simulink model "tank"  (R2019b)
settings: Solver=ode45  StartTime=0.0  StopTime=inf  RelTol=1e-3  EnableMultiTasking=on
model workspace (MAT data in the model file):
  PLC_IP_Address = 'localhost'
libraries: sh_lib x74, nesl_utility x46, fl_lib x40, dspnetwork x33
(part 1 of 3)
settings Model: EnablePacing=on  PacingRate=0.100000  Creator=Rishabh  LastModifiedBy=jrsma
settings DataIOCC: LimitDataPoints=on  SaveFormat=Array  SignalLoggingSaveFormat=ModelDataLogs  ReturnWorkspaceOutputs=off
settings OptimizationCC: ExpressionDepthLimit=2147483647  InitFltsAndDblsToZero=on  LifeSpan=inf
settings DebuggingCC: UnderspecifiedInitializationDetection=Classic  MergeDetectMultiDrivingBlocksExec=none  SolverPrmCheckMsg=warning  FcnCallInpInsideContextMsg=warning  AllowSymbolicDim=off  StateNameClashWarn=warning  SFUnexpectedBacktrackingDiag=warning  SFNoUnconditionalDefaultTransitionDiag=warning  SFExecutionAtInitializationDiag=none  ArithmeticOperatorsInVariantConditions=warning
settings HardwareCC: ProdBitPerPointer=32  ProdBitPerSizeT=32  ProdBitPerPtrDiffT=32  ProdLargestAtomicFloat=None  ProdIntDivRoundTo=Undefined  ProdEndianess=Unspecified  ProdWordSize=32  ProdHWDeviceType=32-bit Generic
settings ModelReferenceCC: PropagateSignalLabelsOutOfModel=off
settings SFSimCC: SimUseLocalCustomCode=off  CustomCodeUndefinedFunction=UseInterfaceOnly
settings RTWCC: RTWUseLocalCustomCode=off
settings CodeAppCC: StateflowObjectComments=on
settings GRTTargetCC: TargetLangStandard=C89/C90 (ANSI)  CombineOutputUpdateFcns=off  GRTInterface=on
settings ConfigComp: CovMetricSettings=dw  CovHtmlReporting=on  CovSaveCumulativeToWorkspaceVar=on  CovSaveSingleToWorkspaceVar=on  CovExternalEMLEnable=off
settings SimscapeCC: SimscapeNormalizeSystem=off

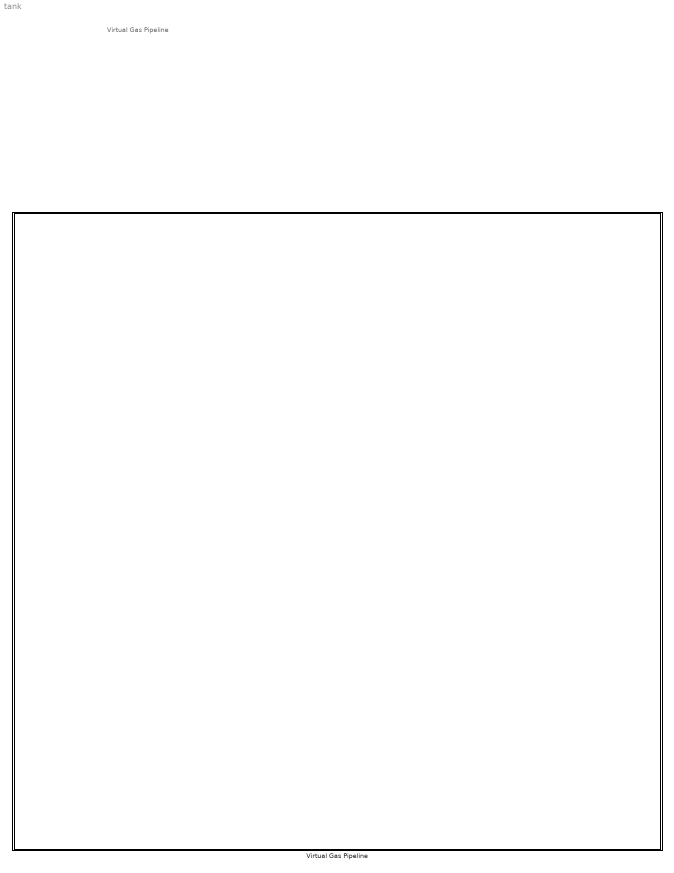
== system tank ==
  note: Virtual Gas Pipeline
  "Virtual Gas Pipeline " : Subsystem

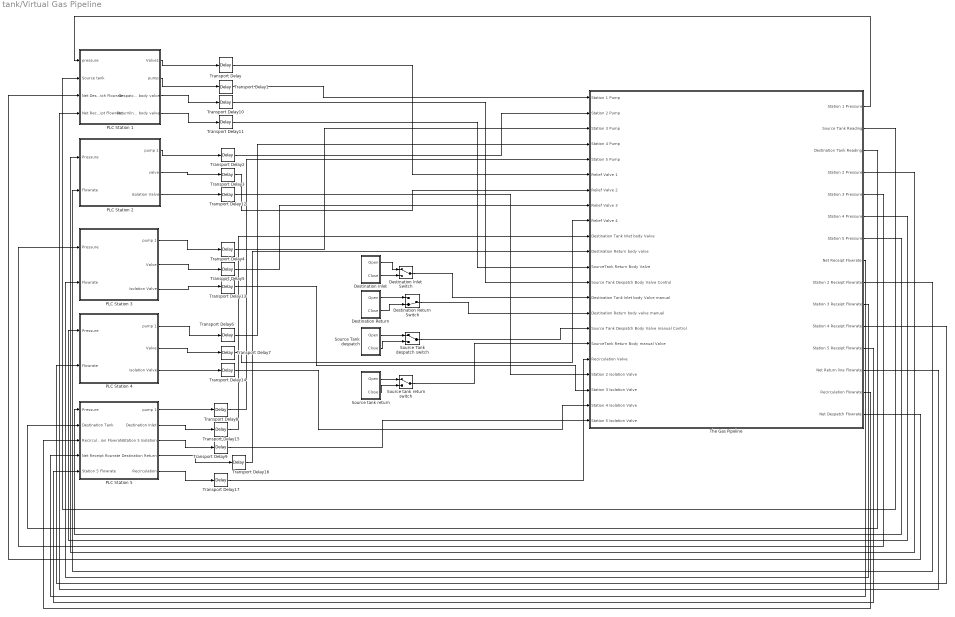
== system tank/Virtual Gas Pipeline  ==
  "  PLC Station 2" : Subsystem  TreatAsAtomicUnit=on
  " PLC Station 1" : Subsystem  TreatAsAtomicUnit=on
  Destination Inlet : Subsystem
  Destination Inlet Switch : ManualSwitch
  Destination Return : Subsystem
  Destination Return Switch : ManualSwitch  CurrentSetting=0
  PLC Station 3 : Subsystem  TreatAsAtomicUnit=on
  PLC Station 4 : Subsystem  TreatAsAtomicUnit=on
  PLC Station 5 : Subsystem  TreatAsAtomicUnit=on
  Source Tank despatch : Subsystem
  Source Tank despatch switch : ManualSwitch
  "Source tank return " : Subsystem
  Source tank return switch : ManualSwitch
  The Gas Pipeline : Subsystem
  Transport Delay{,1..17} (18 alike) : TransportDelay  DelayTime=0.00002
  wires:
  The Gas Pipeline/1(Station 1 Pressure) -> " PLC Station 1"/1(pressure)
  PLC Station 3/1(pump 1) -> Transport Delay4/1
  PLC Station 3/2(Valve) -> Transport Delay5/1
  "  PLC Station 2"/2(valve) -> Transport Delay3/1
  PLC Station 4/2(Valve) -> Transport Delay7/1
  PLC Station 5/1(pump 1) -> Transport Delay8/1
  "  PLC Station 2"/1(pump 1) -> Transport Delay2/1
  " PLC Station 1"/2("pump ") -> Transport Delay1/1
  " PLC Station 1"/1(Valve1) -> Transport Delay/1
  PLC Station 4/1(pump 1) -> Transport Delay6/1
  The Gas Pipeline/2(Source Tank Reading) -> " PLC Station 1"/2(Source tank)
  The Gas Pipeline/3(Destination Tank Reading) -> PLC Station 5/2(Destination Tank)
  Destination Inlet/1(Open) -> Destination Inlet Switch/1
  Destination Inlet/2("Close ") -> Destination Inlet Switch/2
  Destination Inlet Switch/1 -> The Gas Pipeline/14(Destination Tank Inlet body Valve manual)
  Destination Return/1(Open) -> Destination Return Switch/1
  Destination Return/2(Close) -> Destination Return Switch/2
  Destination Return Switch/1 -> The Gas Pipeline/15(Destination Return body valve manual)
  Source Tank despatch/1(Open) -> Source Tank despatch switch/1
  Source Tank despatch/2(Close) -> Source Tank despatch switch/2
  Source Tank despatch switch/1 -> The Gas Pipeline/16(Source Tank Despatch Body Valve manual Control)
  "Source tank return "/1(Open) -> Source tank return switch/1
  "Source tank return "/2(Close) -> Source tank return switch/2
  Source tank return switch/1 -> The Gas Pipeline/17(SourceTank Return Body manual Valve)
  The Gas Pipeline/7(Station 5 Pressure) -> PLC Station 5/1("Pressure ")
  The Gas Pipeline/6(Station 4 Pressure) -> PLC Station 4/1("Pressure ")
  The Gas Pipeline/5(Station 3 Pressure) -> PLC Station 3/1("Pressure ")
  The Gas Pipeline/4(Station 2 Pressure) -> "  PLC Station 2"/1(Pressure)
  Transport Delay/1 -> The Gas Pipeline/6(Relief Valve 1)
  Transport Delay1/1 -> The Gas Pipeline/1(Station 1 Pump)
  Transport Delay2/1 -> The Gas Pipeline/2("Station 2 Pump ")
  Transport Delay3/1 -> The Gas Pipeline/7(Relief Valve 2)
  Transport Delay4/1 -> The Gas Pipeline/3("Station 3 Pump ")
  Transport Delay5/1 -> The Gas Pipeline/8(Relief Valve 3)
  Transport Delay6/1 -> The Gas Pipeline/4("Station 4 Pump ")
  Transport Delay8/1 -> The Gas Pipeline/5(Station 5 Pump)
  Transport Delay7/1 -> The Gas Pipeline/9(Relief Valve 4)
  The Gas Pipeline/15(Net Despatch Flowrate) -> " PLC Station 1"/3(Net Despatch Flowrate)
  The Gas Pipeline/9(Station 2 Receipt Flowrate) -> "  PLC Station 2"/2(Flowrate)
  The Gas Pipeline/10(Station 3 Receipt Flowrate) -> PLC Station 3/2(Flowrate)
  The Gas Pipeline/11(Station 4 Receipt Flowrate) -> PLC Station 4/2(Flowrate)
  The Gas Pipeline/13(Net Return line Flowrate) -> " PLC Station 1"/4(Net Receipt Flowrate)
  " PLC Station 1"/3(Despatch body valve) -> Transport Delay10/1
  " PLC Station 1"/4(Returnline body valve) -> Transport Delay11/1
  Transport Delay10/1 -> The Gas Pipeline/13(Source Tank Despatch Body Valve Control)
  Transport Delay11/1 -> The Gas Pipeline/12(SourceTank Return Body Valve)
  "  PLC Station 2"/3(Isolation Valve) -> Transport Delay12/1
  Transport Delay12/1 -> The Gas Pipeline/19(Station 2 Isolation Valve)
  PLC Station 3/3(Isolation Valve) -> Transport Delay13/1
  Transport Delay13/1 -> The Gas Pipeline/20(Station 3 Isolation Valve)
  PLC Station 4/3(Isolation Valve) -> Transport Delay14/1
  Transport Delay14/1 -> The Gas Pipeline/21(Station 4 Isolation Valve)
  The Gas Pipeline/8(Net Receipt Flowrate) -> PLC Station 5/4(Net Receipt flowrate)
  The Gas Pipeline/12(Station 5 Receipt Flowrate) -> PLC Station 5/5(Station 5 Flowrate)
  The Gas Pipeline/14(Recirculation Flowrate) -> PLC Station 5/3(Recirculation Flowrate)
  PLC Station 5/2(Destination Inlet) -> Transport Delay15/1
  PLC Station 5/3(Station 5 Isolation) -> Transport Delay9/1
  PLC Station 5/4(Destination Return) -> Transport Delay16/1
  PLC Station 5/5(Recirculation) -> Transport Delay17/1
  Transport Delay15/1 -> The Gas Pipeline/10(Destination Tank Inlet body Valve)
  Transport Delay9/1 -> The Gas Pipeline/22(Station 5 Isolation Valve)
  Transport Delay16/1 -> The Gas Pipeline/11(Destination Return body valve)
  Transport Delay17/1 -> The Gas Pipeline/18(Recirculation Valve)

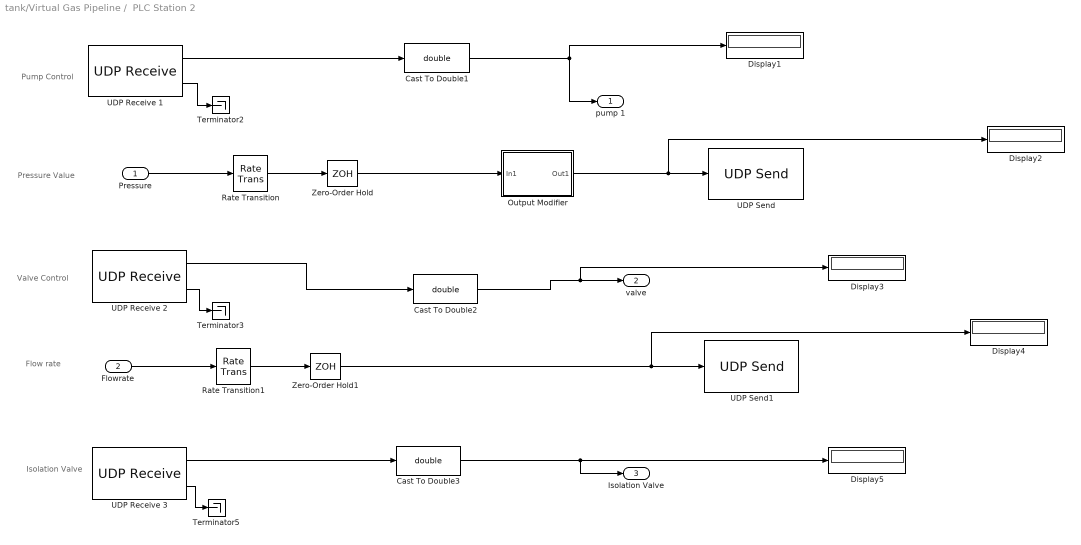
== system tank/Virtual Gas Pipeline /  PLC Station 2 ==
  note: Isolation Valve
  note: Flow rate
  note: Valve Control
  note: Pump Control
  note: Pressure Value
  Pressure : Inport
  Flowrate : Inport  Port=2
  Cast To Double1 : DataTypeConversion  OutDataTypeStr=double
  Cast To Double2 : DataTypeConversion  OutDataTypeStr=double
  Cast To Double3 : DataTypeConversion  OutDataTypeStr=double
  Display{1..5} (5 alike) : Display
  Output Modifier : Subsystem
  Rate Transition : RateTransition
  Rate Transition1 : RateTransition
  Terminator2 : Terminator
  Terminator3 : Terminator
  Terminator5 : Terminator
  UDP Receive 1 : dspnetwork/UDP Receive  localURL='0.0.0.0'  localPort=20001  remoteURL='0.0.0.0'  remotePort=-1  recvBufferSize=2  dims=1  signalDatatype=uint16  isComplex=off  isVarSize=off  showBlockingTime=on  blockingTime=0  sampletime=0.01  blockPlatform=LINUX
      settings: SourceProductName=Simulink
  UDP Receive 2 : dspnetwork/UDP Receive  localURL='0.0.0.0'  localPort=20003  remoteURL='0.0.0.0'  remotePort=-1  recvBufferSize=2  dims=1  signalDatatype=uint16  isComplex=off  isVarSize=off  showBlockingTime=on  blockingTime=0  sampletime=0.01  blockPlatform=LINUX
      settings: SourceProductName=Simulink
  UDP Receive 3 : dspnetwork/UDP Receive  localURL='0.0.0.0'  localPort=20005  remoteURL='0.0.0.0'  remotePort=-1  recvBufferSize=2  dims=1  signalDatatype=uint16  isComplex=off  isVarSize=off  showBlockingTime=on  blockingTime=0  sampletime=0.01  blockPlatform=LINUX
      settings: SourceProductName=Simulink
  UDP Send : dspnetwork/UDP Send  remoteURL=PLC_IP_Address  remotePort=20002  localURL='255.255.255.255'  localPortSource=Automatically determine  localPort=-1  sampletime=-1  blockPlatform=LINUX  separateLengthPort=0
      settings: SourceProductName=Simulink
  UDP Send1 : dspnetwork/UDP Send  remoteURL=PLC_IP_Address  remotePort=20004  localURL='255.255.255.255'  localPortSource=Automatically determine  localPort=-1  sampletime=-1  blockPlatform=LINUX  separateLengthPort=0
      settings: SourceProductName=Simulink
  Zero-Order Hold : ZeroOrderHold  SampleTime=0.1
  Zero-Order Hold1 : ZeroOrderHold  SampleTime=0.1
  pump 1 : Outport  PortDimensions=1
  valve : Outport  Port=2  PortDimensions=1
  Isolation Valve : Outport  Port=3  PortDimensions=1
  wires:
  UDP Receive 1/2 -> Terminator2/1
  UDP Receive 2/1 -> Cast To Double2/1
  UDP Receive 2/2 -> Terminator3/1
  Cast To Double2/1 -> Display3/1, valve/1
  Rate Transition/1 -> Zero-Order Hold/1
  Pressure/1 -> Rate Transition/1
  Cast To Double1/1 -> pump 1/1, Display1/1
  Zero-Order Hold/1 -> Output Modifier/1(In1)
  Output Modifier/1(Out1) -> Display2/1, UDP Send/1
  Rate Transition1/1 -> Zero-Order Hold1/1
  Flowrate/1 -> Rate Transition1/1
  Zero-Order Hold1/1 -> Display4/1, UDP Send1/1
  UDP Receive 3/1 -> Cast To Double3/1
  UDP Receive 3/2 -> Terminator5/1
  Cast To Double3/1 -> Isolation Valve/1, Display5/1
  UDP Receive 1/1 -> Cast To Double1/1

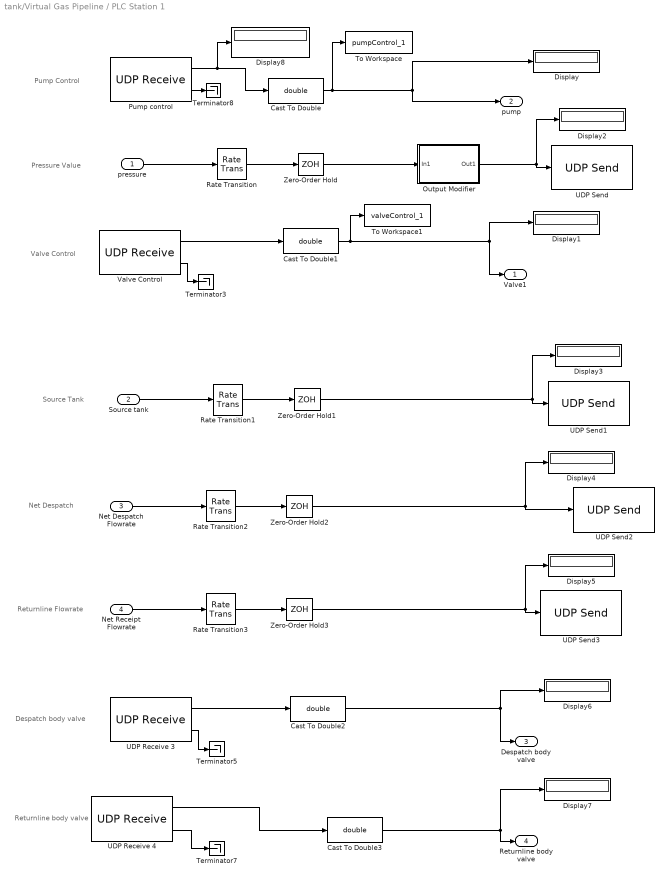
== system tank/Virtual Gas Pipeline / PLC Station 1 ==
  note: Despatch body valve
  note: Returnline body valve
  note: Returnline Flowrate
  note: Net Despatch
  note: Source Tank
  note: Valve Control
  note: Pump Control
  note: Pressure Value
  pressure : Inport
  Source tank : Inport  Port=2
  Net Despatch Flowrate : Inport  Port=3
  Net Receipt Flowrate : Inport  Port=4
  Cast To Double{,1..3} (4 alike) : DataTypeConversion  OutDataTypeStr=double
  Display{,1..8} (9 alike) : Display
  Output Modifier : Subsystem
  Pump control : dspnetwork/UDP Receive  localURL='0.0.0.0'  localPort=10001  remoteURL='0.0.0.0'  remotePort=-1  recvBufferSize=2  dims=1  signalDatatype=uint16  isComplex=off  isVarSize=off  showBlockingTime=on  blockingTime=0  sampletime=0.01  blockPlatform=LINUX
      settings: SourceProductName=Simulink
  Rate Transition{,1..3} (4 alike) : RateTransition
  Terminator{3,5,7..8} (4 alike) : Terminator
  To Workspace : ToWorkspace  VariableName=pumpControl_1  SaveFormat=Timeseries  SampleTime=-1
  To Workspace1 : ToWorkspace  VariableName=valveControl_1  SaveFormat=Timeseries  SampleTime=-1
  UDP Receive 3 : dspnetwork/UDP Receive  localURL='0.0.0.0'  localPort=10007  remoteURL='0.0.0.0'  remotePort=-1  recvBufferSize=2  dims=1  signalDatatype=uint16  isComplex=off  isVarSize=off  showBlockingTime=on  blockingTime=0  sampletime=0.01  blockPlatform=LINUX
      settings: SourceProductName=Simulink
  UDP Receive 4 : dspnetwork/UDP Receive  localURL='0.0.0.0'  localPort=10008  remoteURL='0.0.0.0'  remotePort=-1  recvBufferSize=2  dims=1  signalDatatype=uint16  isComplex=off  isVarSize=off  showBlockingTime=on  blockingTime=0  sampletime=0.01  blockPlatform=LINUX
      settings: SourceProductName=Simulink
  UDP Send : dspnetwork/UDP Send  remoteURL=PLC_IP_Address  remotePort=10002  localURL='255.255.255.255'  localPortSource=Automatically determine  localPort=-1  sampletime=-1  blockPlatform=LINUX  separateLengthPort=0
      settings: SourceProductName=Simulink
  UDP Send1 : dspnetwork/UDP Send  remoteURL=PLC_IP_Address  remotePort=10004  localURL='255.255.255.255'  localPortSource=Automatically determine  localPort=-1  sampletime=-1  blockPlatform=LINUX  separateLengthPort=0
      settings: SourceProductName=Simulink
  UDP Send2 : dspnetwork/UDP Send  remoteURL=PLC_IP_Address  remotePort=10005  localURL='255.255.255.255'  localPortSource=Automatically determine  localPort=-1  sampletime=-1  blockPlatform=LINUX  separateLengthPort=0
      settings: SourceProductName=Simulink
  UDP Send3 : dspnetwork/UDP Send  remoteURL=PLC_IP_Address  remotePort=10006  localURL='255.255.255.255'  localPortSource=Automatically determine  localPort=-1  sampletime=-1  blockPlatform=LINUX  separateLengthPort=0
      settings: SourceProductName=Simulink
  Valve Control : dspnetwork/UDP Receive  localURL='0.0.0.0'  localPort=10003  remoteURL='0.0.0.0'  remotePort=-1  recvBufferSize=2  dims=1  signalDatatype=uint16  isComplex=off  isVarSize=off  showBlockingTime=on  blockingTime=0  sampletime=0.01  blockPlatform=LINUX
      settings: SourceProductName=Simulink
  Zero-Order Hold{,1..3} (4 alike) : ZeroOrderHold  SampleTime=0.1
  Valve1 : Outport  PortDimensions=1
  "pump " : Outport  Port=2  PortDimensions=1
  Despatch body valve : Outport  Port=3  PortDimensions=1
  Returnline body valve : Outport  Port=4  PortDimensions=1
  wires:
  Valve Control/1 -> Cast To Double1/1
  Valve Control/2 -> Terminator3/1
  Rate Transition/1 -> Zero-Order Hold/1
  pressure/1 -> Rate Transition/1
  Cast To Double1/1 -> To Workspace1/1, Valve1/1, Display1/1
  Output Modifier/1(Out1) -> UDP Send/1, Display2/1
  Zero-Order Hold/1 -> Output Modifier/1(In1)
  Rate Transition1/1 -> Zero-Order Hold1/1
  Source tank/1 -> Rate Transition1/1
  Zero-Order Hold1/1 -> Display3/1, UDP Send1/1
  Rate Transition2/1 -> Zero-Order Hold2/1
  Net Despatch Flowrate/1 -> Rate Transition2/1
  Zero-Order Hold2/1 -> Display4/1, UDP Send2/1
  Rate Transition3/1 -> Zero-Order Hold3/1
  Net Receipt Flowrate/1 -> Rate Transition3/1
  Zero-Order Hold3/1 -> Display5/1, UDP Send3/1
  UDP Receive 3/1 -> Cast To Double2/1
  UDP Receive 3/2 -> Terminator5/1
  Cast To Double2/1 -> Despatch body valve/1, Display6/1
  UDP Receive 4/2 -> Terminator7/1
  Cast To Double3/1 -> Returnline body valve/1, Display7/1
  Pump control/2 -> Terminator8/1
  Pump control/1 -> Cast To Double/1, Display8/1
  Cast To Double/1 -> To Workspace/1, Display/1, "pump "/1
  UDP Receive 4/1 -> Cast To Double3/1

== system tank/Virtual Gas Pipeline /Destination Inlet ==
  Constant : Constant
  Constant1 : Constant  Value=0
  Open : Outport
  "Close " : Outport  Port=2
  wires:
  Constant1/1 -> "Close "/1
  Constant/1 -> Open/1

== system tank/Virtual Gas Pipeline /Destination Return ==
  Constant : Constant
  Constant1 : Constant  Value=0
  Open : Outport
  Close : Outport  Port=2
  wires:
  Constant1/1 -> Close/1
  Constant/1 -> Open/1

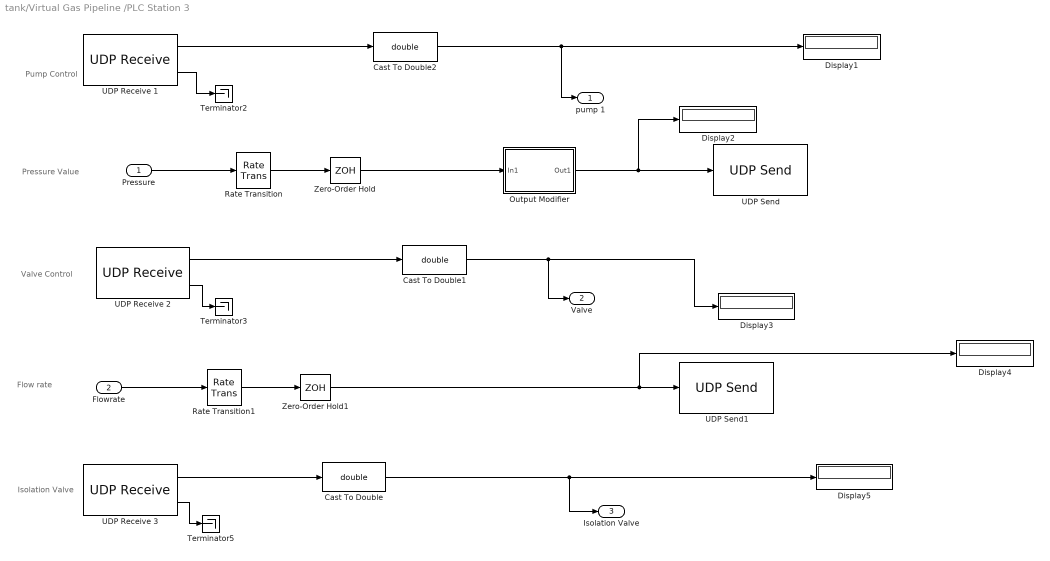
== system tank/Virtual Gas Pipeline /PLC Station 3 ==
  note: Valve Control
  note: Pump Control
  note: Pressure Value
  note: Isolation Valve
  note: Flow rate
  "Pressure " : Inport
  Flowrate : Inport  Port=2
  Cast To Double : DataTypeConversion  OutDataTypeStr=double
  Cast To Double1 : DataTypeConversion  OutDataTypeStr=double
  Cast To Double2 : DataTypeConversion  OutDataTypeStr=double
  Display{1..5} (5 alike) : Display
  Output Modifier : Subsystem
  Rate Transition : RateTransition
  Rate Transition1 : RateTransition
  Terminator2 : Terminator
  Terminator3 : Terminator
  Terminator5 : Terminator
  UDP Receive 1 : dspnetwork/UDP Receive  localURL='0.0.0.0'  localPort=30001  remoteURL='0.0.0.0'  remotePort=-1  recvBufferSize=2  dims=1  signalDatatype=uint16  isComplex=off  isVarSize=off  showBlockingTime=on  blockingTime=0  sampletime=0.01  blockPlatform=LINUX
      settings: SourceProductName=Simulink
  UDP Receive 2 : dspnetwork/UDP Receive  localURL='0.0.0.0'  localPort=30003  remoteURL='0.0.0.0'  remotePort=-1  recvBufferSize=2  dims=1  signalDatatype=uint16  isComplex=off  isVarSize=off  showBlockingTime=on  blockingTime=0  sampletime=0.01  blockPlatform=LINUX
      settings: SourceProductName=Simulink
  UDP Receive 3 : dspnetwork/UDP Receive  localURL='0.0.0.0'  localPort=30005  remoteURL='0.0.0.0'  remotePort=-1  recvBufferSize=2  dims=1  signalDatatype=uint16  isComplex=off  isVarSize=off  showBlockingTime=on  blockingTime=0  sampletime=0.01  blockPlatform=LINUX
      settings: SourceProductName=Simulink
  UDP Send : dspnetwork/UDP Send  remoteURL=PLC_IP_Address  remotePort=30002  localURL='255.255.255.255'  localPortSource=Automatically determine  localPort=-1  sampletime=-1  blockPlatform=LINUX  separateLengthPort=0
      settings: SourceProductName=Simulink
  UDP Send1 : dspnetwork/UDP Send  remoteURL=PLC_IP_Address  remotePort=30004  localURL='255.255.255.255'  localPortSource=Automatically determine  localPort=-1  sampletime=-1  blockPlatform=LINUX  separateLengthPort=0
      settings: SourceProductName=Simulink
  Zero-Order Hold : ZeroOrderHold  SampleTime=0.1
  Zero-Order Hold1 : ZeroOrderHold  SampleTime=0.1
  pump 1 : Outport  PortDimensions=1
  Valve : Outport  Port=2  PortDimensions=1
  Isolation Valve : Outport  Port=3  PortDimensions=1
  wires:
  UDP Receive 1/2 -> Terminator2/1
  UDP Receive 2/2 -> Terminator3/1
  Cast To Double1/1 -> Valve/1, Display3/1
  Cast To Double2/1 -> pump 1/1, Display1/1
  Rate Transition/1 -> Zero-Order Hold/1
  "Pressure "/1 -> Rate Transition/1
  Zero-Order Hold/1 -> Output Modifier/1(In1)
  Output Modifier/1(Out1) -> Display2/1, UDP Send/1
  Rate Transition1/1 -> Zero-Order Hold1/1
  Flowrate/1 -> Rate Transition1/1
  Zero-Order Hold1/1 -> Display4/1, UDP Send1/1
  UDP Receive 3/2 -> Terminator5/1
  Cast To Double/1 -> Isolation Valve/1, Display5/1
  UDP Receive 1/1 -> Cast To Double2/1
  UDP Receive 2/1 -> Cast To Double1/1
  UDP Receive 3/1 -> Cast To Double/1

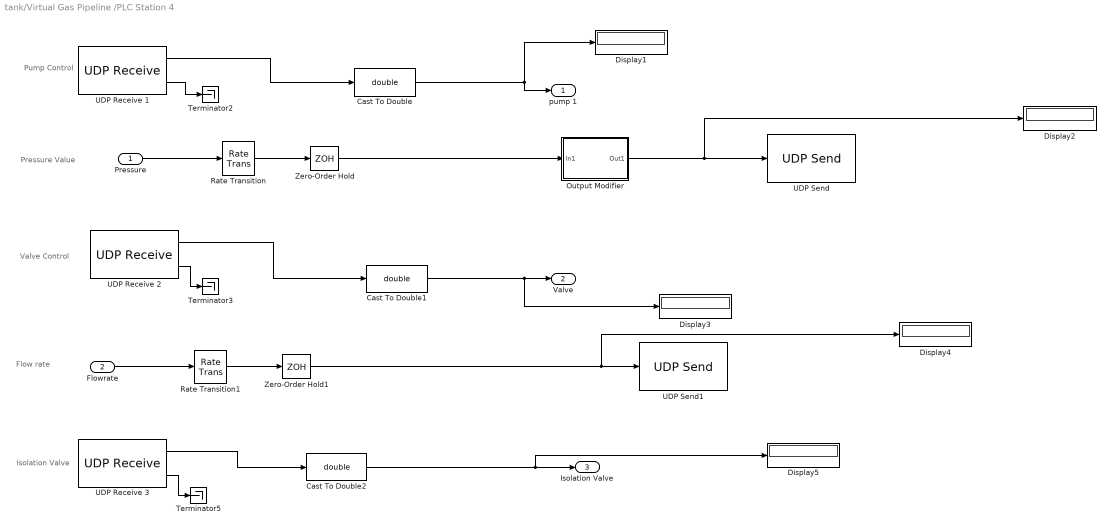
== system tank/Virtual Gas Pipeline /PLC Station 4 ==
  note: Valve Control
  note: Pump Control
  note: Pressure Value
  note: Isolation Valve
  note: Flow rate
  "Pressure " : Inport
  Flowrate : Inport  Port=2
  Cast To Double : DataTypeConversion  OutDataTypeStr=double
  Cast To Double1 : DataTypeConversion  OutDataTypeStr=double
  Cast To Double2 : DataTypeConversion  OutDataTypeStr=double
  Display{1..5} (5 alike) : Display
  Output Modifier : Subsystem
  Rate Transition : RateTransition
  Rate Transition1 : RateTransition
  Terminator2 : Terminator
  Terminator3 : Terminator
  Terminator5 : Terminator
  UDP Receive 1 : dspnetwork/UDP Receive  localURL='0.0.0.0'  localPort=40001  remoteURL='0.0.0.0'  remotePort=-1  recvBufferSize=2  dims=1  signalDatatype=uint16  isComplex=off  isVarSize=off  showBlockingTime=on  blockingTime=0  sampletime=0.01  blockPlatform=LINUX
      settings: SourceProductName=Simulink
  UDP Receive 2 : dspnetwork/UDP Receive  localURL='0.0.0.0'  localPort=40003  remoteURL='0.0.0.0'  remotePort=-1  recvBufferSize=2  dims=1  signalDatatype=uint16  isComplex=off  isVarSize=off  showBlockingTime=on  blockingTime=0  sampletime=0.01  blockPlatform=LINUX
      settings: SourceProductName=Simulink
  UDP Receive 3 : dspnetwork/UDP Receive  localURL='0.0.0.0'  localPort=40005  remoteURL='0.0.0.0'  remotePort=-1  recvBufferSize=2  dims=1  signalDatatype=uint16  isComplex=off  isVarSize=off  showBlockingTime=on  blockingTime=0  sampletime=0.01  blockPlatform=LINUX
      settings: SourceProductName=Simulink
  UDP Send : dspnetwork/UDP Send  remoteURL=PLC_IP_Address  remotePort=40002  localURL='255.255.255.255'  localPortSource=Automatically determine  localPort=-1  sampletime=-1  blockPlatform=LINUX  separateLengthPort=0
      settings: SourceProductName=Simulink
  UDP Send1 : dspnetwork/UDP Send  remoteURL=PLC_IP_Address  remotePort=40004  localURL='255.255.255.255'  localPortSource=Automatically determine  localPort=-1  sampletime=-1  blockPlatform=LINUX  separateLengthPort=0
      settings: SourceProductName=Simulink
  Zero-Order Hold : ZeroOrderHold  SampleTime=0.1
  Zero-Order Hold1 : ZeroOrderHold  SampleTime=0.1
  pump 1 : Outport  PortDimensions=1
  Valve : Outport  Port=2  PortDimensions=1
  Isolation Valve : Outport  Port=3  PortDimensions=1
  wires:
  UDP Receive 1/2 -> Terminator2/1
  UDP Receive 2/1 -> Cast To Double1/1
  UDP Receive 2/2 -> Terminator3/1
  Cast To Double1/1 -> Display3/1, Valve/1
  Cast To Double/1 -> pump 1/1, Display1/1
  UDP Receive 1/1 -> Cast To Double/1
  Rate Transition/1 -> Zero-Order Hold/1
  "Pressure "/1 -> Rate Transition/1
  Zero-Order Hold/1 -> Output Modifier/1(In1)
  Output Modifier/1(Out1) -> Display2/1, UDP Send/1
  Rate Transition1/1 -> Zero-Order Hold1/1
  Flowrate/1 -> Rate Transition1/1
  Zero-Order Hold1/1 -> Display4/1, UDP Send1/1
  UDP Receive 3/1 -> Cast To Double2/1
  UDP Receive 3/2 -> Terminator5/1
  Cast To Double2/1 -> Display5/1, Isolation Valve/1

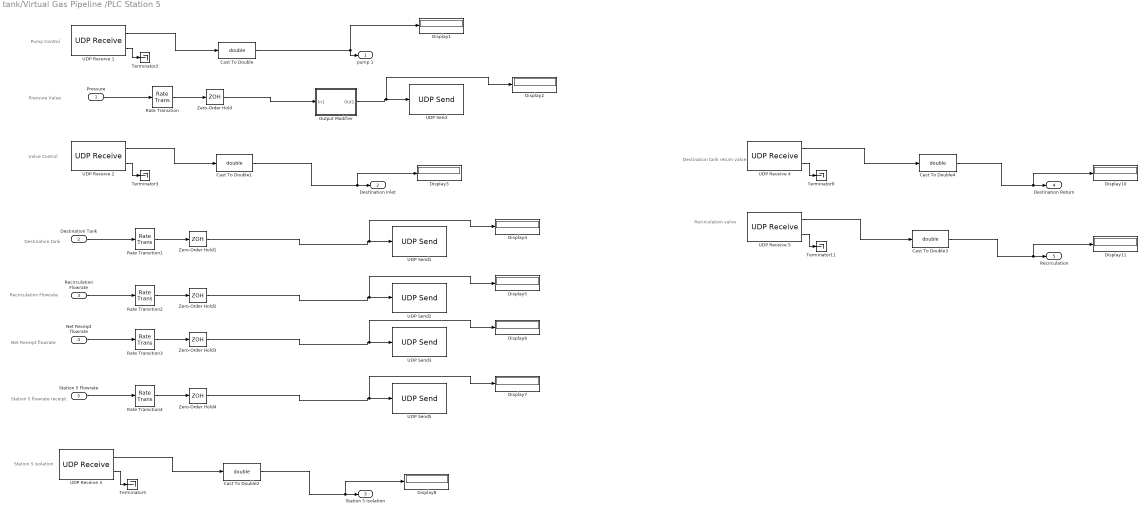
== system tank/Virtual Gas Pipeline /PLC Station 5 ==
  note: Recirculation valve
  note: Destination tank return valve
  note: Station 5 Isolation
  note: Net Receipt flowrate
  note: Recirculation Flowrate
  note: Destination tank
  note: Valve Control
  note: Pump Control
  note: Pressure Value
  note: Station 5 flowrate receipt
  "Pressure " : Inport
  Destination Tank : Inport  Port=2
  Recirculation Flowrate : Inport  Port=3
  Net Receipt flowrate : Inport  Port=4
  Station 5 Flowrate : Inport  Port=5
  Cast To Double{,1..4} (5 alike) : DataTypeConversion  OutDataTypeStr=double
  Display{1..8,10..11} (10 alike) : Display
  Output Modifier : Subsystem
  Rate Transition{,1..4} (5 alike) : RateTransition
  Terminator{2..3,5,9,11} (5 alike) : Terminator
  UDP Receive 1 : dspnetwork/UDP Receive  localURL='0.0.0.0'  localPort=50001  remoteURL='0.0.0.0'  remotePort=-1  recvBufferSize=2  dims=1  signalDatatype=uint16  isComplex=off  isVarSize=off  showBlockingTime=on  blockingTime=0  sampletime=0.01  blockPlatform=LINUX
      settings: SourceProductName=Simulink
  UDP Receive 2 : dspnetwork/UDP Receive  localURL='0.0.0.0'  localPort=50003  remoteURL='0.0.0.0'  remotePort=-1  recvBufferSize=2  dims=1  signalDatatype=uint16  isComplex=off  isVarSize=off  showBlockingTime=on  blockingTime=0  sampletime=0.01  blockPlatform=LINUX
      settings: SourceProductName=Simulink
  UDP Receive 3 : dspnetwork/UDP Receive  localURL='0.0.0.0'  localPort=50008  remoteURL='0.0.0.0'  remotePort=-1  recvBufferSize=2  dims=1  signalDatatype=uint16  isComplex=off  isVarSize=off  showBlockingTime=on  blockingTime=0  sampletime=0.01  blockPlatform=LINUX
      settings: SourceProductName=Simulink
  UDP Receive 4 : dspnetwork/UDP Receive  localURL='0.0.0.0'  localPort=5009  remoteURL='0.0.0.0'  remotePort=-1  recvBufferSize=2  dims=1  signalDatatype=uint16  isComplex=off  isVarSize=off  showBlockingTime=on  blockingTime=0  sampletime=0.01  blockPlatform=LINUX
      settings: SourceProductName=Simulink
  UDP Receive 5 : dspnetwork/UDP Receive  localURL='0.0.0.0'  localPort=50010  remoteURL='0.0.0.0'  remotePort=-1  recvBufferSize=2  dims=1  signalDatatype=uint16  isComplex=off  isVarSize=off  showBlockingTime=on  blockingTime=0  sampletime=0.01  blockPlatform=LINUX
      settings: SourceProductName=Simulink
  UDP Send : dspnetwork/UDP Send  remoteURL=PLC_IP_Address  remotePort=50002  localURL='255.255.255.255'  localPortSource=Automatically determine  localPort=-1  sampletime=-1  blockPlatform=LINUX  separateLengthPort=0
      settings: SourceProductName=Simulink
  UDP Send1 : dspnetwork/UDP Send  remoteURL=PLC_IP_Address  remotePort=50004  localURL='255.255.255.255'  localPortSource=Automatically determine  localPort=-1  sampletime=-1  blockPlatform=LINUX  separateLengthPort=0
      settings: SourceProductName=Simulink
  UDP Send2 : dspnetwork/UDP Send  remoteURL=PLC_IP_Address  remotePort=50005  localURL='255.255.255.255'  localPortSource=Automatically determine  localPort=-1  sampletime=-1  blockPlatform=LINUX  separateLengthPort=0
      settings: SourceProductName=Simulink
  UDP Send3 : dspnetwork/UDP Send  remoteURL=PLC_IP_Address  remotePort=50006  localURL='255.255.255.255'  localPortSource=Automatically determine  localPort=-1  sampletime=-1  blockPlatform=LINUX  separateLengthPort=0
      settings: SourceProductName=Simulink
  UDP Send5 : dspnetwork/UDP Send  remoteURL=PLC_IP_Address  remotePort=50007  localURL='255.255.255.255'  localPortSource=Automatically determine  localPort=-1  sampletime=-1  blockPlatform=LINUX  separateLengthPort=0
      settings: SourceProductName=Simulink
  Zero-Order Hold{,1..4} (5 alike) : ZeroOrderHold  SampleTime=0.1
  pump 1 : Outport  PortDimensions=1
  Destination Inlet : Outport  Port=2  PortDimensions=1
  Station 5 Isolation : Outport  Port=3  PortDimensions=1
  Destination Return : Outport  Port=4  PortDimensions=1
  Recirculation : Outport  Port=5  PortDimensions=1
  wires:
  UDP Receive 1/2 -> Terminator2/1
  UDP Receive 2/2 -> Terminator3/1
  Cast To Double1/1 -> Display3/1, Destination Inlet/1
  Cast To Double/1 -> pump 1/1, Display1/1
  Rate Transition/1 -> Zero-Order Hold/1
  "Pressure "/1 -> Rate Transition/1
  Output Modifier/1(Out1) -> Display2/1, UDP Send/1
  Zero-Order Hold/1 -> Output Modifier/1(In1)
  Rate Transition1/1 -> Zero-Order Hold1/1
  Destination Tank/1 -> Rate Transition1/1
  Zero-Order Hold1/1 -> Display4/1, UDP Send1/1
  Rate Transition2/1 -> Zero-Order Hold2/1
  Recirculation Flowrate/1 -> Rate Transition2/1
  Zero-Order Hold2/1 -> Display5/1, UDP Send2/1
  Rate Transition3/1 -> Zero-Order Hold3/1
  Net Receipt flowrate/1 -> Rate Transition3/1
  Zero-Order Hold3/1 -> Display6/1, UDP Send3/1
  Rate Transition4/1 -> Zero-Order Hold4/1
  Station 5 Flowrate/1 -> Rate Transition4/1
  Zero-Order Hold4/1 -> Display7/1, UDP Send5/1
  UDP Receive 3/1 -> Cast To Double2/1
  UDP Receive 3/2 -> Terminator5/1
  Cast To Double2/1 -> Display8/1, Station 5 Isolation/1
  UDP Receive 4/1 -> Cast To Double4/1
  UDP Receive 4/2 -> Terminator9/1
  Cast To Double4/1 -> Display10/1, Destination Return/1
  UDP Receive 5/1 -> Cast To Double3/1
  UDP Receive 5/2 -> Terminator11/1
  Cast To Double3/1 -> Display11/1, Recirculation/1
  UDP Receive 1/1 -> Cast To Double/1
  UDP Receive 2/1 -> Cast To Double1/1

== system tank/Virtual Gas Pipeline /Source Tank despatch ==
  Constant : Constant
  Constant1 : Constant  Value=0
  Open : Outport
  Close : Outport  Port=2
  wires:
  Constant1/1 -> Close/1
  Constant/1 -> Open/1

== system tank/Virtual Gas Pipeline /Source tank return  ==
  Constant : Constant
  Constant1 : Constant  Value=0
  Open : Outport
  Close : Outport  Port=2
  wires:
  Constant1/1 -> Close/1
  Constant/1 -> Open/1

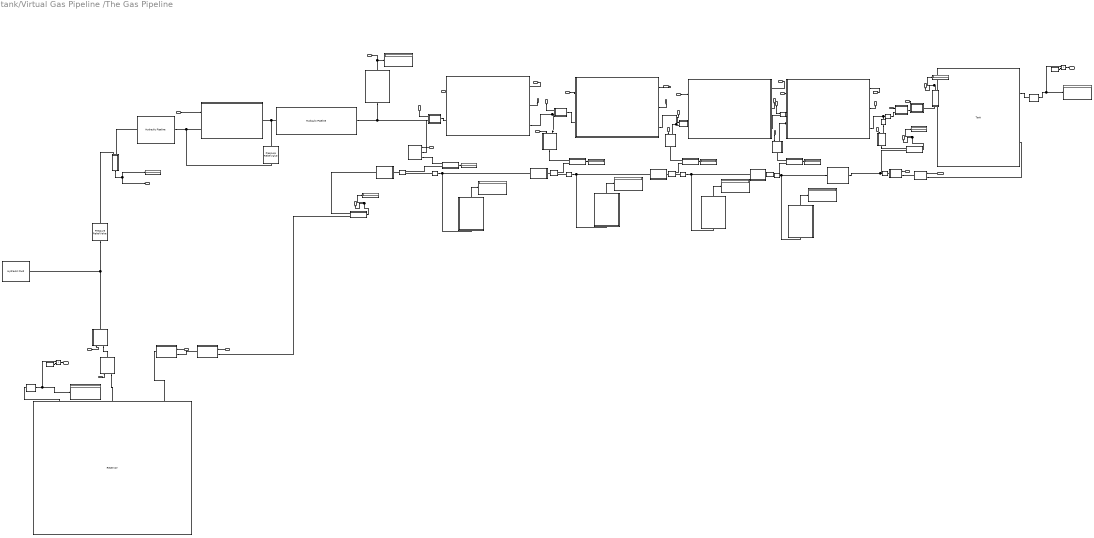
== system tank/Virtual Gas Pipeline /The Gas Pipeline ==
  note: Refrigerated Gas Pipeline Simulation
      |
      | This is a model of a Virtual gas pipeline. This is specifically designed to simulate the behaviour of a pipeline used in transferring Liquified gases like Ammonia,Butane,Propane.etc. Provisions have been made to have the Preecooling and normal cargo transfer operation setup.
  Station 1 Pump : Inport
  "Station 2 Pump " : Inport  Port=2
  "Station 3 Pump " : Inport  Port=3
  "Station 4 Pump " : Inport  Port=4
  Station 5 Pump : Inport  Port=5
  Relief Valve 1 : Inport  Port=6
  Relief Valve 2 : Inport  Port=7
  Relief Valve 3 : Inport  Port=8
  Relief Valve 4 : Inport  Port=9
  Destination Tank Inlet body Valve : Inport  Port=10
  Destination Return body valve : Inport  Port=11
  SourceTank Return Body Valve : Inport  Port=12
  Source Tank Despatch Body Valve Control : Inport  Port=13
  Destination Tank Inlet body Valve manual : Inport  Port=14
  Destination Return body valve manual : Inport  Port=15
  Source Tank Despatch Body Valve manual Control : Inport  Port=16
  SourceTank Return Body manual Valve : Inport  Port=17
  Recirculation Valve : Inport  Port=18
  Station 2 Isolation Valve : Inport  Port=19
  Station 3 Isolation Valve : Inport  Port=20
  Station 4 Isolation Valve : Inport  Port=21
  Station 5 Isolation Valve : Inport  Port=22
  Ball Valve1 : Subsystem
  Ball Valve2 : Subsystem
  Ball Valve3 : Subsystem
  Ball Valve4 : Subsystem
  Ball Valve5 : Subsystem
  Ball Valve6 : Subsystem
  Ball Valve7 : Subsystem
  Constant : Constant  Value=10
  Constant1 : Constant  Value=10
  "Destination tank " : sh_lib/Low-Pressure Blocks/Tank  press=0 Pa  level_spec=1  tank_area=314 m^2  fluid_volume_tab=[ 0 0.0028 0.0065 0.0114 0.0176 0.0252 0.0344 0.0436 0.0512 0.0574 0.0623 0.066 0.0688 0.0707 0.07199999999999999 0.0727 ] m^3  fluid_level_tab=[ 0 0.02 0.04 0.06 0.08 0.1 0.12 0.14 0.16 0.18 0.2 0.22 0.24 0.26 0.28 0.3 ] m  interp_method=1  extrap_method=1  pipe_diam=0.02 m  loss_coeff=1.2  g=9.80665 m/s^2  min_level=1e-3 m  fluid_level_check=0  volume_specify=on  volume_priority=High  volume=30 m^3  volume_nominal_specify=off  volume_nominal_unit=l  volume_nominal_value=1  level_specify=off  level_priority=None  level=0.025 m  level_nominal_specify=off  level_nominal_unit=m  level_nominal_value=1  pipe_diam_A=6 m  loss_coeff_A=1.2  height_B=0.5 m  pipe_diam_B=16 m  loss_coeff_B=1.2  height_C=0.8 m  pipe_diam_C=0.02 m  loss_coeff_C=1.2
      settings: SourceProductName=Simscape Fluids  SourceProductBaseCode=SH  InternalSimscapePortConfiguration="{\"Bottom\":[],\"Left\":[{\"id\":\"B\",\"label\":\"B\",\"type\":\"foundation.hydraulic.hydraulic\"}],\"Right\":[{\"id\":\"V\",\"label\":\"V\",\"type\":\"output\"},{\"id\":\"A\",\"label\":\"A\",\"type\":\"foundation.hydraulic.hydraulic\"}],\"Top\":[]}"
  Display1 : Display
  First 3 Km pipeline segment : sh_lib/Pipelines/Hydraulic Pipeline  cs_type=1  d_in=16 in  area=1e-04 m^2  D_h=0.0112 m  s_factor=64  length=3000 m  length_ad=3000 m  roughness=1.5e-3 m  Re_lam=2e+03  Re_turb=4e+03  wall_type=1  pr_r_coef=2e-12 m/Pa  time_const=0.01 s  k_sh=1.4  initial_pressure=0 Pa
      settings: SourceProductName=Simscape Fluids  SourceProductBaseCode=SH  InternalSimscapePortConfiguration="{\"Bottom\":[],\"Left\":[{\"id\":\"A\",\"label\":\"A\",\"type\":\"foundation.hydraulic.hydraulic\"}],\"Right\":[{\"id\":\"B\",\"label\":\"B\",\"type\":\"foundation.hydraulic.hydraulic\"}],\"Top\":[]}"
  Flow Measurement (KL/Hr) : Subsystem
  Flow Measurement (KL/Hr)1 : Subsystem
  Flow Measurement (KL/Hr)2 : Subsystem
  Flow Measurement (KL/Hr)3 : Subsystem
  Flow Measurement (KL/Hr)4 : Subsystem
  Flow Measurement (KL/Hr)5 : Subsystem
  Flow Measurement (KL/Hr)6 : Subsystem
  Flow Measurement (KL/Hr)7 : Subsystem
  Flow rate Display{,1..7} (8 alike) : Display
  Hydraulic Fluid : sh_lib/Hydraulic Utilities/Hydraulic Fluid  DataSource=1  SelFluid=20  SysTemp=30  TrapAir=0.005  ViscDerFactor=1  range_error=1
      settings: SourceProductName=Simscape Fluids
  NRV{1..7} (7 alike) : sh_lib/Valves/Pressure Control Valves/Pressure Relief Valve  valve_area_spec=1  p_diff_TLU=[30.15e5 : 15e3 : 31.35e5] Pa  area_TLU=[1 : 1 : 9] .* 1e-5 m^2  area_max=500 in^2  pres_set=0.001 bar  reg_range=5 psi  C_d=0.7  A_leak=1e-12 m^2  lam_spec=2  B_lam=0.999  Re_cr=12  dynamic=0  tau=0.1 s  area_init=1e-12 m^2
      settings: SourceProductName=Simscape Fluids  SourceProductBaseCode=SH  InternalSimscapePortConfiguration="{\"Bottom\":[],\"Left\":[{\"id\":\"A\",\"label\":\"A\",\"type\":\"foundation.hydraulic.hydraulic\"}],\"Right\":[{\"id\":\"B\",\"label\":\"B\",\"type\":\"foundation.hydraulic.hydraulic\"}],\"Top\":[]}"
  PS-Simulink Converter : nesl_utility/PS-Simulink Converter  PhysicalDomain=network_engine_domain  SubClassName=ps_output  LeftPortType=input  RightPortType=output  PseudoPeriodic=off  Frequencies=[]  Unit=1  AffineConversion=off
  PS-Simulink Converter1 : nesl_utility/PS-Simulink Converter  PhysicalDomain=network_engine_domain  SubClassName=ps_output  LeftPortType=input  RightPortType=output  PseudoPeriodic=off  Frequencies=[]  Unit=1  AffineConversion=off
  Pressure Sensor : Subsystem
  Pressure Sensor Display{,5..8} (5 alike) : Display
  Pressure Sensor1 : Subsystem
  Pressure Sensor2 : Subsystem
  Pressure Sensor3 : Subsystem
  Pressure Sensor4 : Subsystem
  Primary Pumping station (500 kl/hr) : Subsystem
  Product : Product
  Product1 : Product
  Protection against High Pressure : sh_lib/Valves/Pressure Control Valves/Pressure Relief Valve  valve_area_spec=1  p_diff_TLU=[30.15e5 : 15e3 : 31.35e5] Pa  area_TLU=[1 : 1 : 9] .* 1e-5 m^2  area_max=157 in^2  pres_set=150 psi  reg_range=5 psi  C_d=0.7  A_leak=1e-12 m^2  lam_spec=2  B_lam=0.999  Re_cr=12  dynamic=0  tau=0.1 s  area_init=1e-12 m^2
      settings: SourceProductName=Simscape Fluids  SourceProductBaseCode=SH  InternalSimscapePortConfiguration="{\"Bottom\":[],\"Left\":[{\"id\":\"A\",\"label\":\"A\",\"type\":\"foundation.hydraulic.hydraulic\"}],\"Right\":[{\"id\":\"B\",\"label\":\"B\",\"type\":\"foundation.hydraulic.hydraulic\"}],\"Top\":[]}"
  Protection against High Pressure1 : sh_lib/Valves/Pressure Control Valves/Pressure Relief Valve  valve_area_spec=1  p_diff_TLU=[30.15e5 : 15e3 : 31.35e5] Pa  area_TLU=[1 : 1 : 9] .* 1e-5 m^2  area_max=157 in^2  pres_set=.1 bar  reg_range=5 psi  C_d=0.7  A_leak=1e-12 m^2  lam_spec=2  B_lam=0.999  Re_cr=12  dynamic=0  tau=0.1 s  area_init=1e-12 m^2
      settings: SourceProductName=Simscape Fluids  SourceProductBaseCode=SH  InternalSimscapePortConfiguration="{\"Bottom\":[],\"Left\":[{\"id\":\"A\",\"label\":\"A\",\"type\":\"foundation.hydraulic.hydraulic\"}],\"Right\":[{\"id\":\"B\",\"label\":\"B\",\"type\":\"foundation.hydraulic.hydraulic\"}],\"Top\":[]}"
  Recirculation valve : Subsystem
  "Relief Valve 1 " : Subsystem
  Reservoir : sh_lib/Hydraulic Utilities/Reservoir  press=0 bar  init_volume=500 m^3  ret_diam=6 in  loss_coeff=1
      settings: SourceProductName=Simscape Fluids  SourceProductBaseCode=SH  InternalSimscapePortConfiguration="{\"Bottom\":[],\"Left\":[{\"id\":\"V\",\"label\":\"V\",\"type\":\"output\"},{\"id\":\"P\",\"label\":\"P\",\"type\":\"foundation.hydraulic.hydraulic\"},{\"id\":\"R\",\"label\":\"R\",\"type\":\"foundation.hydraulic.hydraulic\"}],\"Right\":[],\"Top\":[]}"
  Return line : Subsystem
  "Return line 1 " : Subsystem
  Return line1 : Subsystem
  Return line2 : Subsystem
  Return line3 : Subsystem
  Source Return line body valve : Subsystem
  Source Return line body valve1 : Subsystem
  Source Tank Body Valve : Subsystem
  Source Tank Body Valve1 : Subsystem
  Station 2 (With 3km pipeline) : Subsystem
  Station 2 inlet valve : Subsystem
  Station 3 (With 3km pipeline) : Subsystem
  Station 3 inlet valve : Subsystem
  Station 4 (With 3km pipeline) : Subsystem
  Station 4 inlet valve : Subsystem
  Station 5 (With 3km pipeline) : Subsystem
  Station 5 inlet valve : Subsystem
  T-junction{,1..3} (4 alike) : sh_lib/Local Hydraulic Resistances/T-junction  main_diam=6 in  branch_diam=6 in  kp_ab=1.12  kp_ba=1.12  kp_aa1=1.36  kp_a1a=1.65  kp_a1b=1.6  kp_ba1=1.8  lam_spec=2  B_lam=0.999  Re_cr=120
      settings: SourceProductName=Simscape Fluids  SourceProductBaseCode=SH  InternalSimscapePortConfiguration="{\"Bottom\":[],\"Left\":[{\"id\":\"A\",\"label\":\"A\",\"type\":\"foundation.hydraulic.hydraulic\"},{\"id\":\"A1\",\"label\":\"A1\",\"type\":\"foundation.hydraulic.hydraulic\"}],\"Right\":[{\"id\":\"B\",\"label\":\"B\",\"type\":\"foundation.hydraulic.hydraulic\"}],\"Top\":[]}"
  Tank Level : Display
  Tank to primary pump pipeline : sh_lib/Pipelines/Hydraulic Pipeline  cs_type=1  d_in=16 in  area=1e-04 m^2  D_h=0.0112 m  s_factor=64  length=50 m  length_ad=1 m  roughness=1.5e-05 m  Re_lam=2e+03  Re_turb=4e+03  wall_type=1  pr_r_coef=2e-12 m/Pa  time_const=0.01 s  k_sh=1.4  initial_pressure=0 Pa
      settings: SourceProductName=Simscape Fluids  SourceProductBaseCode=SH  InternalSimscapePortConfiguration="{\"Bottom\":[],\"Left\":[{\"id\":\"A\",\"label\":\"A\",\"type\":\"foundation.hydraulic.hydraulic\"}],\"Right\":[{\"id\":\"B\",\"label\":\"B\",\"type\":\"foundation.hydraulic.hydraulic\"}],\"Top\":[]}"
  Station 1 Pressure : Outport
  Source Tank Reading : Outport  Port=2
  Destination Tank Reading : Outport  Port=3
  Station 2 Pressure : Outport  Port=4
  Station 3 Pressure : Outport  Port=5
  Station 4 Pressure : Outport  Port=6
  Station 5 Pressure : Outport  Port=7
  Net Receipt Flowrate : Outport  Port=8
  Station 2 Receipt Flowrate : Outport  Port=9
  Station 3 Receipt Flowrate : Outport  Port=10
  Station 4 Receipt Flowrate : Outport  Port=11
  Station 5 Receipt Flowrate : Outport  Port=12
  Net Return line Flowrate : Outport  Port=13
  Recirculation Flowrate : Outport  Port=14
  Net Despatch Flowrate : Outport  Port=15
  wires:
  Relief Valve 3/1 -> Ball Valve2/1(Relief Valve Control)
  Relief Valve 4/1 -> Ball Valve3/1(Relief Valve Control)
  Destination Tank Inlet body Valve/1 -> Ball Valve4/1(valve)
  PS-Simulink Converter1/1 -> Product/1, Tank Level/1
  Destination Return body valve/1 -> Ball Valve6/1(valve)
  Station 1 Pump/1 -> Primary Pumping station (500 kl/hr)/1(Pump 1 Control)
  "Station 2 Pump "/1 -> Station 2 (With 3km pipeline)/1(Station 2 Pump)
  "Station 4 Pump "/1 -> Station 4 (With 3km pipeline)/1("Station 4 Pump ")
  Station 5 Pump/1 -> Station 5 (With 3km pipeline)/1(Station 5 pump)
  Relief Valve 1/1 -> "Relief Valve 1 "/1(Relief Valve 1 Control)
  Pressure Sensor/1(" Display") -> Station 1 Pressure/1, Pressure Sensor Display/1
  Source Tank Despatch Body Valve Control/1 -> Source Tank Body Valve/1(valve)
  SourceTank Return Body Valve/1 -> Source Return line body valve/1(valve)
  "Station 3 Pump "/1 -> Station 3 (With 3km pipeline)/1(Station 3 Pump)
  Relief Valve 2/1 -> Ball Valve1/1(Relief Valve Control)
  Destination Tank Inlet body Valve manual/1 -> Ball Valve5/1(valve)
  Destination Return body valve manual/1 -> Ball Valve7/1(valve)
  Source Tank Despatch Body Valve manual Control/1 -> Source Tank Body Valve1/1(valve)
  SourceTank Return Body manual Valve/1 -> Source Return line body valve1/1(valve)
  Pressure Sensor1/1(" Display") -> Pressure Sensor Display5/1
  Pressure Sensor2/1(" Display") -> Pressure Sensor Display6/1
  Pressure Sensor3/1(" Display") -> Pressure Sensor Display7/1
  Pressure Sensor4/1(" Display") -> Pressure Sensor Display8/1
  Station 2 (With 3km pipeline)/1(Station 2 Pressure) -> Station 2 Pressure/1
  Station 3 (With 3km pipeline)/1(Station 3 Pressure) -> Station 3 Pressure/1
  Station 4 (With 3km pipeline)/1(Station 4 Pressure) -> Station 4 Pressure/1
  Station 5 (With 3km pipeline)/1(Station 5 Pressure) -> Station 5 Pressure/1
  Constant/1 -> Product/2
  Product/1 -> Source Tank Reading/1
  PS-Simulink Converter/1 -> Product1/1, Display1/1
  Constant1/1 -> Product1/2
  Product1/1 -> Destination Tank Reading/1
  Recirculation Valve/1 -> Recirculation valve/1(valve)
  Station 2 Isolation Valve/1 -> Station 2 inlet valve/1(valve)
  Station 3 Isolation Valve/1 -> Station 3 inlet valve/1(valve)
  Station 4 Isolation Valve/1 -> Station 4 inlet valve/1(valve)
  Station 5 Isolation Valve/1 -> Station 5 inlet valve/1(valve)
  Flow Measurement (KL/Hr)/1(Display out) -> Net Receipt Flowrate/1, Flow rate Display/1
  Station 2 (With 3km pipeline)/2(Station 2 Flowrate) -> Station 2 Receipt Flowrate/1
  Station 3 (With 3km pipeline)/2(Station 3 Flowrate) -> Station 3 Receipt Flowrate/1
  Station 4 (With 3km pipeline)/2(Station 4 Flowrate) -> Station 4 Receipt Flowrate/1
  Station 5 (With 3km pipeline)/2(Station 5 Flowrate) -> Station 5 Receipt Flowrate/1
  Flow Measurement (KL/Hr)1/1(Display out) -> Net Return line Flowrate/1, Flow rate Display1/1
  Flow Measurement (KL/Hr)2/1(Display out) -> Recirculation Flowrate/1, Flow rate Display2/1
  Flow Measurement (KL/Hr)3/1(Display out) -> Net Despatch Flowrate/1, Flow rate Display3/1
  Flow Measurement (KL/Hr)4/1(Display out) -> Flow rate Display4/1
  Flow Measurement (KL/Hr)5/1(Display out) -> Flow rate Display5/1
  Flow Measurement (KL/Hr)6/1(Display out) -> Flow rate Display6/1
  Flow Measurement (KL/Hr)7/1(Display out) -> Flow rate Display7/1
  connections:
  Source Tank Body Valve/RConn1 -- Protection against High Pressure1/LConn1 -- Hydraulic Fluid/RConn1
  Station 3 inlet valve/LConn1 -- Ball Valve1/LConn1 -- Station 2 (With 3km pipeline)/RConn1
  "Destination tank "/RConn1 -- PS-Simulink Converter/LConn1
  Return line3/LConn1 -- Flow Measurement (KL/Hr)2/LConn2 -- NRV1/RConn1
  Return line3/RConn1 -- Pressure Sensor4/LConn1 -- NRV2/LConn1
  First 3 Km pipeline segment/LConn1 -- Protection against High Pressure/LConn1 -- Primary Pumping station (500 kl/hr)/RConn1
  Tank to primary pump pipeline/RConn1 -- Protection against High Pressure/RConn1 -- Primary Pumping station (500 kl/hr)/LConn1
  PS-Simulink Converter1/LConn1 -- Reservoir/LConn1
  Pressure Sensor/LConn1 -- First 3 Km pipeline segment/RConn1 -- "Relief Valve 1 "/LConn1 -- Station 2 inlet valve/LConn1
  Pressure Sensor1/LConn1 -- Return line/RConn1 -- NRV7/LConn1
  Station 4 inlet valve/LConn1 -- Ball Valve2/LConn1 -- Station 3 (With 3km pipeline)/RConn1
  T-junction/RConn1 -- "Return line 1 "/LConn1
  Station 5 inlet valve/RConn1 -- Ball Valve3/LConn1 -- Station 5 (With 3km pipeline)/LConn1
  T-junction1/RConn1 -- Return line/LConn1
  T-junction2/RConn1 -- Return line1/LConn1
  Return line2/RConn1 -- NRV3/LConn1 -- Pressure Sensor3/LConn1
  T-junction3/RConn1 -- Return line2/LConn1
  Ball Valve4/RConn1 -- Ball Valve5/LConn1
  Ball Valve6/LConn1 -- Ball Valve7/RConn1
  Ball Valve7/LConn1 -- "Destination tank "/RConn2
  Source Tank Body Valve/LConn1 -- Source Tank Body Valve1/RConn1
  Source Tank Body Valve1/LConn1 -- Reservoir/LConn2
  Source Return line body valve1/LConn1 -- Source Return line body valve/RConn1
  Source Return line body valve1/RConn1 -- Reservoir/LConn3
  NRV4/RConn1 -- Ball Valve4/LConn1
  NRV5/LConn1 -- Station 5 (With 3km pipeline)/RConn1 -- NRV4/LConn1
  Return line1/RConn1 -- NRV6/LConn1 -- Pressure Sensor2/LConn1
  NRV5/RConn1 -- Recirculation valve/LConn1
  Station 2 inlet valve/RConn1 -- Station 2 (With 3km pipeline)/LConn1
  Station 3 inlet valve/RConn1 -- Station 3 (With 3km pipeline)/LConn1
  Station 4 inlet valve/RConn1 -- Station 4 (With 3km pipeline)/LConn1
  Station 4 (With 3km pipeline)/RConn1 -- Station 5 inlet valve/LConn1
  Flow Measurement (KL/Hr)/LConn1 -- Ball Valve5/RConn1
  Flow Measurement (KL/Hr)/LConn2 -- "Destination tank "/LConn1
  "Return line 1 "/RConn1 -- Flow Measurement (KL/Hr)1/LConn1
  Source Return line body valve/LConn1 -- Flow Measurement (KL/Hr)1/LConn2
  Recirculation valve/RConn1 -- Flow Measurement (KL/Hr)2/LConn1
  Flow Measurement (KL/Hr)3/LConn1 -- Protection against High Pressure1/RConn1
  Flow Measurement (KL/Hr)3/LConn2 -- Tank to primary pump pipeline/LConn1
  "Relief Valve 1 "/LConn2 -- Flow Measurement (KL/Hr)4/LConn1
  Flow Measurement (KL/Hr)4/LConn2 -- T-junction/LConn1
  Ball Valve1/RConn1 -- Flow Measurement (KL/Hr)5/LConn1
  Flow Measurement (KL/Hr)5/LConn2 -- T-junction1/LConn1
  Flow Measurement (KL/Hr)6/LConn1 -- Ball Valve2/RConn1
  Flow Measurement (KL/Hr)6/LConn2 -- T-junction2/LConn1
  Flow Measurement (KL/Hr)7/LConn1 -- Ball Valve3/RConn1
  Flow Measurement (KL/Hr)7/LConn2 -- T-junction3/LConn1
  NRV1/LConn1 -- Ball Valve6/RConn1
  NRV2/RConn1 -- T-junction3/LConn2
  NRV3/RConn1 -- T-junction2/LConn2
  NRV6/RConn1 -- T-junction1/LConn2
  NRV7/RConn1 -- T-junction/LConn2

== system tank/Virtual Gas Pipeline /  PLC Station 2/Output Modifier ==
  In1 : Inport
  Add : Sum
  Constant : Constant  Value=0.001
  Constant1 : Constant  Value=100
  Product : Product
  Out1 : Outport
  wires:
  Constant/1 -> Product/2
  In1/1 -> Product/1
  Add/1 -> Out1/1
  Product/1 -> Add/1
  Constant1/1 -> Add/2

== system tank/Virtual Gas Pipeline / PLC Station 1/Output Modifier ==
  In1 : Inport
  Add : Sum
  Constant : Constant  Value=0.001
  Constant1 : Constant  Value=100
  Product : Product
  Out1 : Outport
  wires:
  Constant/1 -> Product/2
  In1/1 -> Product/1
  Add/1 -> Out1/1
  Product/1 -> Add/1
  Constant1/1 -> Add/2

== system tank/Virtual Gas Pipeline /PLC Station 3/Output Modifier ==
  In1 : Inport
  Add : Sum
  Constant : Constant  Value=0.001
  Constant1 : Constant  Value=100
  Product : Product
  Out1 : Outport
  wires:
  Constant/1 -> Product/2
  In1/1 -> Product/1
  Add/1 -> Out1/1
  Product/1 -> Add/1
  Constant1/1 -> Add/2

== system tank/Virtual Gas Pipeline /PLC Station 4/Output Modifier ==
  In1 : Inport
  Add : Sum
  Constant : Constant  Value=0.001
  Constant1 : Constant  Value=100
  Product : Product
  Out1 : Outport
  wires:
  Constant/1 -> Product/2
  In1/1 -> Product/1
  Add/1 -> Out1/1
  Product/1 -> Add/1
  Constant1/1 -> Add/2

== system tank/Virtual Gas Pipeline /PLC Station 5/Output Modifier ==
  In1 : Inport
  Add : Sum
  Constant : Constant  Value=0.001
  Constant1 : Constant  Value=100
  Product : Product
  Out1 : Outport
  wires:
  Constant/1 -> Product/2
  In1/1 -> Product/1
  Add/1 -> Out1/1
  Product/1 -> Add/1
  Constant1/1 -> Add/2

== system tank/Virtual Gas Pipeline /The Gas Pipeline/Ball Valve1 ==
  Relief Valve Control : Inport
  Ball Valve : sh_lib/Valves/Flow Control Valves/Ball Valve  valve_seat_spec=1  cone_ang=120 deg  d_ball=8 in  d_orif=6 in  x_0=0 m  C_d=0.65  A_leak=1e-12 m^2  lam_spec=2  B_lam=0.999  Re_cr=10  flow_rate_specify=off  flow_rate_priority=None  flow_rate=0.001 m^3/s  flow_rate_nominal_specify=off  flow_rate_nominal_unit=m^3/s  flow_rate_nominal_value=1  pressure_drop_specify=off  pressure_drop_priority=None  pressure_drop=0 Pa  pressure_drop_nominal_specify=off  pressure_drop_nominal_unit=Pa  pressure_drop_nominal_value=1
      settings: SourceProductName=Simscape Fluids  SourceProductBaseCode=SH  InternalSimscapePortConfiguration="{\"Bottom\":[],\"Left\":[{\"id\":\"S\",\"label\":\"S\",\"type\":\"input\"},{\"id\":\"A\",\"label\":\"A\",\"type\":\"foundation.hydraulic.hydraulic\"}],\"Right\":[{\"id\":\"B\",\"label\":\"B\",\"type\":\"foundation.hydraulic.hydraulic\"}],\"Top\":[]}"
  Simulink-PS Converter : nesl_utility/Simulink-PS Converter  PhysicalDomain=network_engine_domain  SubClassName=ps_input  LeftPortType=input  RightPortType=output  PseudoPeriodic=off  Frequencies=[]  NoiseDistribution=none  NoiseParameters=[]  Unit=1  AffineConversion=off  FilteringAndDerivatives=zero  SimscapeFilterOrder=1  InputFilterTimeConstant=0.001  UdotUserProvided=1
  Inlet : PMIOPort  Side=Left
  outlet : PMIOPort  Port=2  Side=Right
  wires:
  Relief Valve Control/1 -> Simulink-PS Converter/1
  connections:
  Simulink-PS Converter/RConn1 -- Ball Valve/LConn1
  Inlet/RConn1 -- Ball Valve/LConn2
  outlet/RConn1 -- Ball Valve/RConn1

== system tank/Virtual Gas Pipeline /The Gas Pipeline/Ball Valve2 ==
  Relief Valve Control : Inport
  Ball Valve : sh_lib/Valves/Flow Control Valves/Ball Valve  valve_seat_spec=1  cone_ang=120 deg  d_ball=8 in  d_orif=6 in  x_0=0 m  C_d=0.65  A_leak=1e-12 m^2  lam_spec=2  B_lam=0.999  Re_cr=10  flow_rate_specify=off  flow_rate_priority=None  flow_rate=0.001 m^3/s  flow_rate_nominal_specify=off  flow_rate_nominal_unit=m^3/s  flow_rate_nominal_value=1  pressure_drop_specify=off  pressure_drop_priority=None  pressure_drop=0 Pa  pressure_drop_nominal_specify=off  pressure_drop_nominal_unit=Pa  pressure_drop_nominal_value=1
      settings: SourceProductName=Simscape Fluids  SourceProductBaseCode=SH  InternalSimscapePortConfiguration="{\"Bottom\":[],\"Left\":[{\"id\":\"S\",\"label\":\"S\",\"type\":\"input\"},{\"id\":\"A\",\"label\":\"A\",\"type\":\"foundation.hydraulic.hydraulic\"}],\"Right\":[{\"id\":\"B\",\"label\":\"B\",\"type\":\"foundation.hydraulic.hydraulic\"}],\"Top\":[]}"
  Simulink-PS Converter : nesl_utility/Simulink-PS Converter  PhysicalDomain=network_engine_domain  SubClassName=ps_input  LeftPortType=input  RightPortType=output  PseudoPeriodic=off  Frequencies=[]  NoiseDistribution=none  NoiseParameters=[]  Unit=1  AffineConversion=off  FilteringAndDerivatives=zero  SimscapeFilterOrder=1  InputFilterTimeConstant=0.001  UdotUserProvided=1
  Inlet : PMIOPort  Side=Left
  outlet : PMIOPort  Port=2  Side=Right
  wires:
  Relief Valve Control/1 -> Simulink-PS Converter/1
  connections:
  Simulink-PS Converter/RConn1 -- Ball Valve/LConn1
  Inlet/RConn1 -- Ball Valve/LConn2
  outlet/RConn1 -- Ball Valve/RConn1

== system tank/Virtual Gas Pipeline /The Gas Pipeline/Ball Valve3 ==
  Relief Valve Control : Inport
  Ball Valve : sh_lib/Valves/Flow Control Valves/Ball Valve  valve_seat_spec=1  cone_ang=120 deg  d_ball=8 in  d_orif=6 in  x_0=0 m  C_d=0.65  A_leak=1e-12 m^2  lam_spec=2  B_lam=0.999  Re_cr=10  flow_rate_specify=off  flow_rate_priority=None  flow_rate=0.001 m^3/s  flow_rate_nominal_specify=off  flow_rate_nominal_unit=m^3/s  flow_rate_nominal_value=1  pressure_drop_specify=off  pressure_drop_priority=None  pressure_drop=0 Pa  pressure_drop_nominal_specify=off  pressure_drop_nominal_unit=Pa  pressure_drop_nominal_value=1
      settings: SourceProductName=Simscape Fluids  SourceProductBaseCode=SH  InternalSimscapePortConfiguration="{\"Bottom\":[],\"Left\":[{\"id\":\"S\",\"label\":\"S\",\"type\":\"input\"},{\"id\":\"A\",\"label\":\"A\",\"type\":\"foundation.hydraulic.hydraulic\"}],\"Right\":[{\"id\":\"B\",\"label\":\"B\",\"type\":\"foundation.hydraulic.hydraulic\"}],\"Top\":[]}"
  Simulink-PS Converter : nesl_utility/Simulink-PS Converter  PhysicalDomain=network_engine_domain  SubClassName=ps_input  LeftPortType=input  RightPortType=output  PseudoPeriodic=off  Frequencies=[]  NoiseDistribution=none  NoiseParameters=[]  Unit=1  AffineConversion=off  FilteringAndDerivatives=zero  SimscapeFilterOrder=1  InputFilterTimeConstant=0.001  UdotUserProvided=1
  Inlet : PMIOPort  Side=Left
  outlet : PMIOPort  Port=2  Side=Right
  wires:
  Relief Valve Control/1 -> Simulink-PS Converter/1
  connections:
  Simulink-PS Converter/RConn1 -- Ball Valve/LConn1
  Inlet/RConn1 -- Ball Valve/LConn2
  outlet/RConn1 -- Ball Valve/RConn1
